simulink model "Conv_LdCalc"  (R2016b)
settings: configuration reference "CodeGenConfigSet" (kept outside this file)
values from neighbouring files (symbols this model uses):
  Conv_trqLd_C = Calibration.Parameter    [init_Conv_LdCalc.m]
  Conv_trqResv_C = Calibration.Parameter    [init_Conv_LdCalc.m]
settings Model: Creator=Wollf  LastModifiedBy=Wollf
settings ConfigSetRef: SourceLocation=Base Workspace

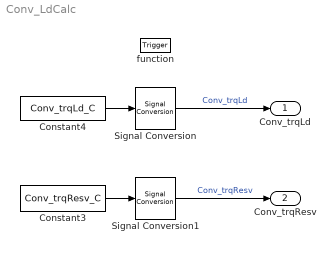
== system Conv_LdCalc ==
  function : TriggerPort  TriggerType=function-call  VariantControl=Variant
  Constant3 : Constant  Value=Conv_trqResv_C  SampleTime=-1
  Constant4 : Constant  Value=Conv_trqLd_C  SampleTime=-1
  Signal Conversion : SignalConversion  OverrideOpt=off
  Signal Conversion1 : SignalConversion  OverrideOpt=off
  Conv_trqLd : Outport  Tag=Nm  Description=Application parameter for torque load from the converter  OutMin=-3000  OutMax=3000  OutDataTypeStr=Trq_Nm
  Conv_trqResv : Outport  Tag=Nm  Description=Torque reserve from the converter  Port=2  OutMin=-3000  OutMax=3000  OutDataTypeStr=Trq_Nm
  wires:
  Constant3/1 -> Signal Conversion1/1
  Constant4/1 -> Signal Conversion/1
  Signal Conversion/1 -> Conv_trqLd/1  "Conv_trqLd"
  Signal Conversion1/1 -> Conv_trqResv/1  "Conv_trqResv"
